simulink model "QR_tuning"  (R2021b)
settings: Solver=ode45  StartTime=0.0  StopTime=5  RelTol=1e-5  EnableMultiTasking=on
values from neighbouring files (symbols this model uses):
  A = [0 0 1 0 ... (first row only)    [main.m]
  B = [0 ... (first row only)    [main.m]
  C = [1 0 0 0 ... (first row only)    [main.m]
  K = K_temp    [plots_assignment2.m]    (also in plots_assignment3.m)
  x_initial = [0 0 0 0]'    [main.m]    (also in tuning.m)
undefined symbols (not defined in the file or in its folder): K_alt
settings Model: Creator=magudelo  LastModifiedBy=Marius
settings SolverCC: AlgebraicLoopSolver=TrustRegion
settings DataIOCC: LimitDataPoints=on  SaveFormat=Array  SignalLoggingSaveFormat=ModelDataLogs  ReturnWorkspaceOutputs=off
settings OptimizationCC: ExpressionDepthLimit=2147483647  LifeSpan=inf
settings DebuggingCC: UnderspecifiedInitializationDetection=Classic  MergeDetectMultiDrivingBlocksExec=none  SolverPrmCheckMsg=warning  FcnCallInpInsideContextMsg=warning  AllowSymbolicDim=off  StateNameClashWarn=warning  SFUnexpectedBacktrackingDiag=warning  SFNoUnconditionalDefaultTransitionDiag=warning  SFExecutionAtInitializationDiag=none  SFMachineParentedDataDiag=warning  ArithmeticOperatorsInVariantConditions=warning
settings HardwareCC: ProdBitPerPointer=32  ProdBitPerSizeT=32  ProdBitPerPtrDiffT=32  ProdLargestAtomicFloat=None  ProdIntDivRoundTo=Undefined  ProdEndianess=Unspecified  ProdWordSize=32  ProdHWDeviceType=32-bit Generic
settings ModelReferenceCC: PropagateSignalLabelsOutOfModel=off
settings SFSimCC: SimUseLocalCustomCode=off  CustomCodeUndefinedFunction=UseInterfaceOnly
settings RTWCC: RTWUseLocalCustomCode=off
settings CodeAppCC: StateflowObjectComments=on
settings GRTTargetCC: TargetLangStandard=C89/C90 (ANSI)  CombineOutputUpdateFcns=off  GRTInterface=on
settings ConfigComp: CovMetricSettings=dw  CovSaveCumulativeToWorkspaceVar=on  CovSaveSingleToWorkspaceVar=on  CovExternalEMLEnable=off

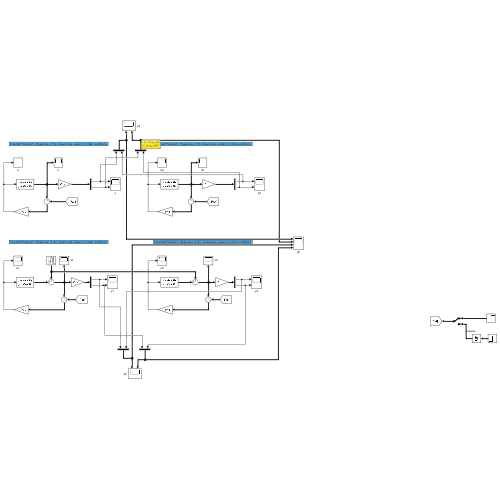
[thumbnail: Simulink's stored preview of the top-level diagram]
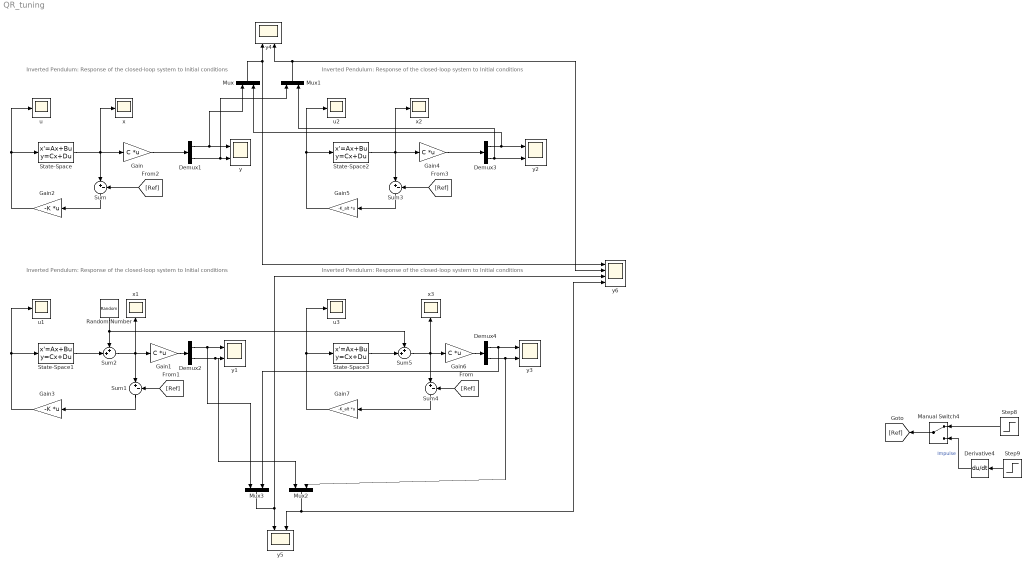
== system QR_tuning ==
  note: Inverted Pendulum: Response of the closed-loop system to Initial conditions
  note: Inverted Pendulum: Response of the closed-loop system to Initial conditions
  note: Inverted Pendulum: Response of the closed-loop system to Initial conditions
  note: Inverted Pendulum: Response of the closed-loop system to Initial conditions
  Demux{1..4} (4 alike) : Demux  Outputs=2
  Derivative4 : Derivative
  Gain{,1,4,6} (4 alike) : Gain  Gain=C  Multiplication=Matrix(K*u)
  Gain2 : Gain  Gain=-K  Multiplication=Matrix(K*u)
  Gain3 : Gain  Gain=-K  Multiplication=Matrix(K*u)
  Gain5 : Gain  Gain=-K_alt  Multiplication=Matrix(K*u)
  Gain7 : Gain  Gain=-K_alt  Multiplication=Matrix(K*u)
  Manual Switch4 : ManualSwitch
  Mux{,1..3} (4 alike) : Mux  Inputs=2
  Random Number : RandomNumber  Mean=[0 0 0 0]  Variance=[0.0005 pi/1800 0 0].^2  SampleTime=0.1
  State-Space{,1..3} (4 alike) : StateSpace  A=A  B=B  C=eye(4)  D=zeros(4,1)  InitialCondition=x_initial
  Step8 : Step  Before=[0 0 0 0]  After=[0.1 0 0 0]  SampleTime=0
  Step9 : Step  Before=[0 0 0 0]  After=[10 0 0 0]  SampleTime=0
  Sum{,1,3..4} (4 alike) : Sum  Inputs=|+-
  Sum2 : Sum  Inputs=++|
  Sum5 : Sum  Inputs=++|
  u{,1..3} (4 alike) : Scope
  x{,1..3} (4 alike) : Scope
  y{,1..5} (6 alike) : Scope  NumInputPorts=2
  y6 : Scope  NumInputPorts=4
  wires:
  Gain/1 -> Demux1/1
  Gain2/1 -> u/1, State-Space/1
  Demux1/1 -> Mux/1, y/1
  Demux1/2 -> Mux1/1, y/2
  Sum/1 -> Gain2/1
  State-Space/1 -> x/1, Sum/1, Gain/1
  Demux2/1 -> Mux3/1, y1/1
  Sum1/1 -> Gain3/1
  Demux2/2 -> Mux2/1, y1/2
  Gain3/1 -> u1/1, State-Space1/1
  Sum2/1 -> Gain1/1, Sum1/1, x1/1
  State-Space1/1 -> Sum2/2
  Gain1/1 -> Demux2/1
  State-Space2/1 -> x2/1, Sum3/1, Gain4/1
  Demux3/1 -> y2/1, Mux/2
  Gain4/1 -> Demux3/1
  Sum3/1 -> Gain5/1
  Demux3/2 -> y2/2, Mux1/2
  Gain5/1 -> u2/1, State-Space2/1
  State-Space3/1 -> Sum5/2
  Gain6/1 -> Demux4/1
  Sum5/1 -> Gain6/1, Sum4/1, x3/1
  Demux4/2 -> y3/2, Mux2/2
  Gain7/1 -> u3/1, State-Space3/1
  Sum4/1 -> Gain7/1
  Random Number/1 -> Sum5/1, Sum2/1
  Demux4/1 -> Mux3/2, y3/1
  Mux/1 -> y6/1, y4/1
  Mux1/1 -> y6/2, y4/2
  Mux3/1 -> y5/1, y6/3
  Mux2/1 -> y6/4, y5/2
  Step9/1 -> Derivative4/1
  Derivative4/1 -> Manual Switch4/2  "Impulse"
  Step8/1 -> Manual Switch4/1
  Manual Switch4/1 -> [Ref]
  [Ref] -> Sum4/2
  [Ref] -> Sum1/2
  [Ref] -> Sum/2
  [Ref] -> Sum3/2
